simulink model "csec_keyconfig_s32k14x"  (Simulink 9.0)
settings: Solver=FixedStepDiscrete  StartTime=0.0  StopTime=10.0  FixedStep=0.1  RelTol=1e-3  EnableMultiTasking=on
PreLoadFcn:
  | mbd_s32k_examples_preload_cbk;
InitFcn:
  | mbd_s32k_consistency_checks(bdroot(gcs));
undefined symbols (not defined in the file): LQFP
libraries: mbd_s32k1xx_ec_toolbox x37, simulink x1
Description:
  | This model presents basic usecases for the CSEc driver.
  | 
  | This application demonstrates how to use:
  | - CSEc_Enable block to enable the CSEc module by partitioning the Flash.
  | - CSEc_Compute_M1M2M3 and CSEc_Load_Key block to configure the MASTER_ECU key and the first user key, using the MASTER_ECU key as an authorization.
  | - CSEc_Encrypt and CSEc_Decrypt blocks to encrypt a plain text and decrypt the cipher text using the first user key.
  | - CSEc_Disable block to disable the CSEc module by erasing of all configured keys (including the MASTER_ECU key) using a Challenge-Authentication process.
  |   This will place the part back into factory status (the CSEc module needs to be enabled again).
  | 
  | Output:
  | - RGB LED is green if the encrypted plain text is the same as the one decrypted.
  | - RGB LED is red if the user key 1 couldn't be updated. This can happened if the counter wasn't increased.
  | - RGB LED is yellow if the CSEc module was disabled successfully.
  | 
  | Note:
  | - The first time when running the example on the board, or after a key erase, this example should be ran from RAM. This is needed because the Flash is partitioned to enable the CSEc module.
  | - The user keys are non-volatile. Once the key was loaded using this example, in order to update it, the counter should be increased.
  | - To disable CSEc module (erase all user keys) set disable_csec_flag to 1.
  | 
  | HW prerequisite:
  | - S32K142EVB-Q100 / S32K144EVB-Q100 / S32K146EVB-Q144 / S32K148EVB-Q144
PostSaveFcn:
  | mbd_s32k_examples_postsave_cbk;
settings Model: Creator=NXP MBDT Team  LastModifiedBy=nxf35172
settings DataIOCC: ExternalInput=off  InitialState=off  LimitDataPoints=on  SaveOutput=off  SignalLogging=off  SaveTime=off
settings OptimizationCC: DefaultParameterBehavior=Inlined  LifeSpan=1
settings DebuggingCC: SolverPrmCheckMsg=warning  InheritedTsInSrcMsg=none  SingleTaskRateTransMsg=error  UnconnectedInputMsg=error  UnconnectedOutputMsg=error  UnconnectedLineMsg=error  AllowSymbolicDim=off  UnknownTsInhSupMsg=error  StateNameClashWarn=warning
settings HardwareCC: ProdLargestAtomicInteger=Long  ProdLargestAtomicFloat=Double  ProdEndianess=LittleEndian  ProdHWDeviceType=ARM Compatible->ARM Cortex
settings SFSimCC: MATLABDynamicMemAlloc=off
settings RTWCC: SystemTargetFile=mbd_s32k.tlc  MakeCommand=mbd_s32k_make_rtw COPY_MDLREF_INCLUDES=0  TemplateMakefile=mbd_s32k.tmf  Description=Model Based Design Toolbox S32K14x Code Generation Target
settings CodeAppCC: IgnoreCustomStorageClasses=off
settings STFCustomTargetCC: CombineOutputUpdateFcns=on  ERTCustomFileBanners=on  SupportContinuousTime=off  SupportNonInlinedSFcns=off  RemoveResetFunc=on  MATLABClassNameForMDSCustomization=Simulink.SoftwareTarget.ERTCustomization  GRTInterface=off  SystemTargetFile=mbd_s32k14.tlc
settings ERTTargetCC: MultiwordLength=2048  ParMdlRefBuildCompliant=off  CompOptLevelCompliant=off  ConcurrentExecutionCompliant=off  ModelStepFunctionPrototypeControlCompliant=off  CPPClassGenCompliant=off  UseToolchainInfoCompliant=off  InlinedParameterPlacement=NonHierarchical  ERTCustomFileTemplate=example_file_process.tlc  ConvertIfToSwitch=off  SuppressUnreachableDefaultCases=off

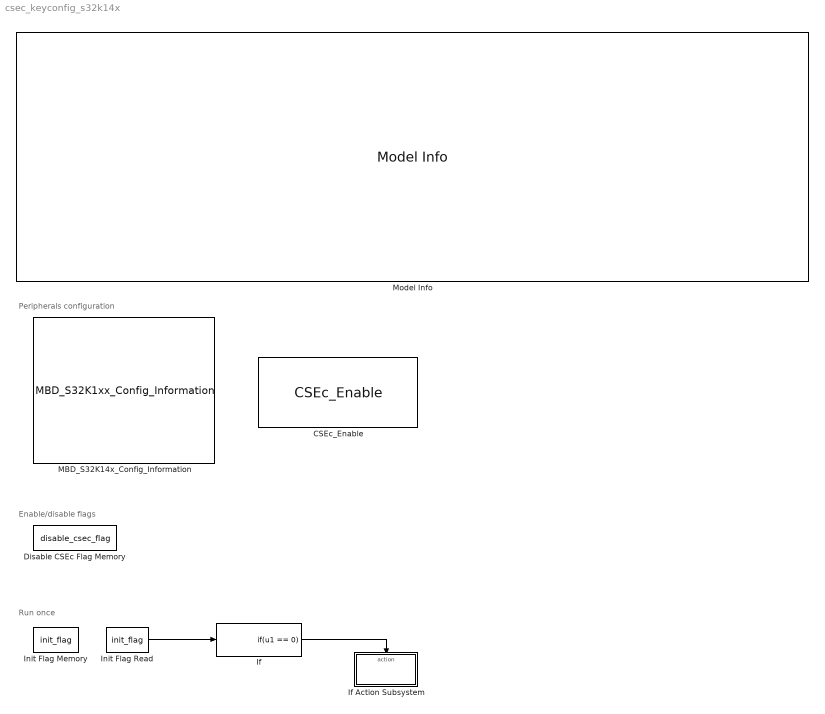
== system csec_keyconfig_s32k14x ==
  note: Enable/disable flags
  note: Peripherals configuration
  note: Run once
  CSEc_Enable : mbd_s32k1xx_ec_toolbox/Core and System Blocks/CSEc Blocks/CSEc_Enable  csec_num_user_keys=20 keys
  Disable CSEc Flag Memory : DataStoreMemory  DataStoreName=disable_csec_flag  ReadBeforeWriteMsg=warning  WriteAfterWriteMsg=warning  WriteAfterReadMsg=warning  InitialValue=1  ShowAdditionalParam=off  OutDataTypeStr=uint32
  If : If  IfExpression=u1 == 0  ShowElse=off
  If Action Subsystem : Subsystem  TreatAsAtomicUnit=on
  Init Flag Memory : DataStoreMemory  DataStoreName=init_flag  ReadBeforeWriteMsg=warning  WriteAfterWriteMsg=warning  WriteAfterReadMsg=warning  ShowAdditionalParam=off  OutDataTypeStr=uint32
  Init Flag Read : DataStoreRead  DataStoreName=init_flag
  MBD_S32K14x_Config_Information : mbd_s32k1xx_ec_toolbox/MBD_S32K1xx_Config_Information  mbdt_ver=0  disp_str=|  config_params=[]  mcu_target_name=S32K144  mcu_target_package=64-LQFP  mcu_target_sram_size=64KB  mcu_system_clock_freq=80  mcu_xtal_freq=External 8  mcu_steptick_timer=LPIT Channel 0  mcu_steptick_prio=15  ds_import_enable=on  target_compiler=GCC  target_memory=SRAM  gcc_target_compile_opts=-mcpu=cortex-m4 -mthumb -mfloat-abi=hard -mfpu=fpv4-sp-d16 -O1 -g -gstrict-dwarf  gcc_target_assemble_opts=-mcpu=cortex-m4 -mthumb -mfloat-abi=hard -mfpu=fpv4-sp-d16 -g  gcc_target_link_opts=-mcpu=cortex-m4 -mthumb -mfloat-abi=hard -mfpu=fpv4-sp-d16  gcc_target_default_lcf=on  gcc_target_user_lcf=S32K144_64_ram.ld  ghs_target_compile_opts=-cpu=cortexm4f -thumb -DARM_MATH_CM4 -fpu=vfpv4_d16 -fsingle -Ogeneral -Wundef -Wimplicit-int -Wshadow -Wtrigraphs --no_commons --gnu_asm -gnu99 -gdwarf-2 -G  ghs_target_assemble_opts=-cpu=cortexm4f -fpu=vfpv4_d16  ghs_target_link_opts=-cpu=cortexm4f -thumb -fpu=vfpv4_d16  ghs_target_default_lcf=off  ghs_target_user_lcf=S32K144_64_ram.ld  iar_target_compile_opts=--cpu=Cortex-M4F --thumb --fpu=VFPv4_sp -Ol -e --debug --dlib_config normal  iar_target_assemble_opts=--cpu Cortex-M4F --thumb --fpu VFPv4_sp  iar_target_link_opts=--no_exceptions --vfe --inline  iar_target_default_lcf=off  iar_target_user_lcf=S32K144_64_ram.icf  pil_download_enable=off  rbl_download_enable=on  rbl_start_delay=5000000  rbl_download_interface=Serial  rbl_restart_request=on  rbl_com_port=Custom  rbl_com_port_custom=COM1  pil_download_rate=57600  pil_opensda_drive=Custom  pil_opensda_drive_custom=D  pil_uart_instance=0  pil_uart_rx=PTA2: [LPUART0_RX | Receive]  pil_uart_tx=PTA3: [LPUART0_TX | Transmit]  FTM_PWM_PcrCheckEnDis=on  FTM_Input_Edge_Inputs_PcrCheckEnDis=on  FTM_Dual_Edge_Inputs_PcrCheckEnDis=on  FTM_Quadrature_Inputs_PcrCheckEnDis=on  FTM_Hall_Sensor_Inputs_PcrCheckEnDis=on  LPTMR_PcrCheckEnDis=on  PIT_PcrCheckEnDis=on  RTC_PcrCheckEnDis=on  FlexCAN_PcrCheckEnDis=on  LIN_PcrCheckEnDis=on  FlexIO_PcrCheckEnDis=on  LPI2C_PcrCheckEnDis=on  LPSPI_PcrCheckEnDis=on  LPUART_PcrCheckEnDis=on  CMP_PcrCheckEnDis=on  GPIO_OutputPcrCheckEnDis=on  GPIO_InputPcrCheckEnDis=on  SBC_PcrCheckEnDis=on  AMMCLIB_PcrCheckEnDis=on  FM_PcrCheckEnDis=on  Profile_PcrCheckEnDis=on  ConfigParams_PcrCheckEnDis=on  ModelRef_PcrCheckEnDis=on  PDB0_PcrCheckEnDis=on  CSEc_PcrCheckEnDis=on  eDMA_PcrCheckEnDis=on  ADC_PcrCheckEnDis=on  WDOG_PcrCheckEnDis=on
      | Target : S32K144-64KB_SRAM
      | Package : 100-pin
      | System clock : 80 MHz
      | XTAL clock : External 8 MHz
      | Compiler : GCC
      | Target Type : SRAM
      | Download Code after build : (COM43, 57600)
      | Step Tick Interrupt Priority : 15
  Model Info : simulink/Model-Wide Utilities/Model Info  Frame=off  DisplayStringWithTags=|  HorizontalTextAlignment=Left  LeftAlignmentValue=0.02
      | Model Name: %<ModelName>
      | 
      | Description: %<Description>
  wires:
  If/1 -> If Action Subsystem/Action
  Init Flag Read/1 -> If/1

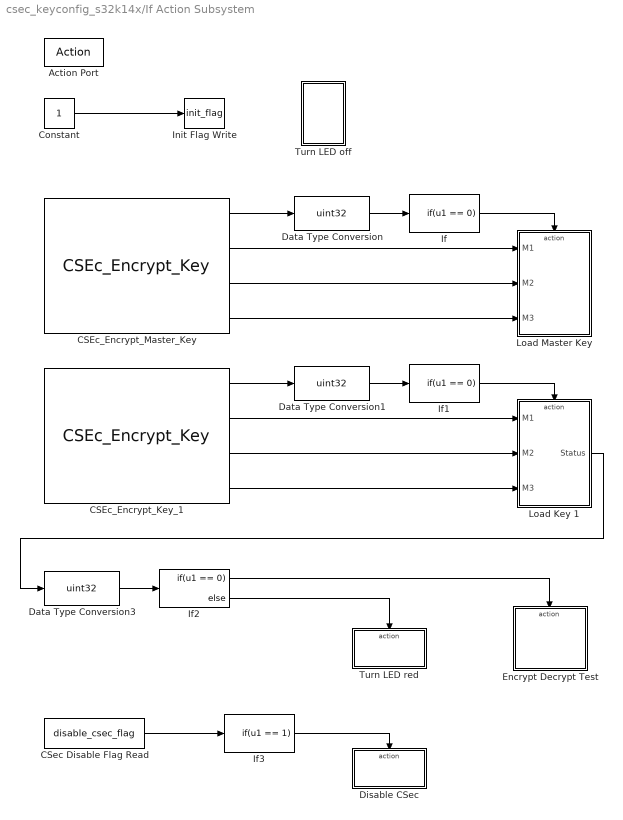
== system csec_keyconfig_s32k14x/If Action Subsystem ==
  Action Port : ActionPort
  CSEc_Encrypt_Key_1 : mbd_s32k1xx_ec_toolbox/Core and System Blocks/CSEc Blocks/CSEc_Encrypt_Key  Priority=3  csec_key_id=KEY_1  csec_key={'0x00', '0x01', '0x02', '0x03', '0x04', '0x05', '0x06', '0x07', '0x08', '0x09', '0x0a', '0x0b', '0x0c', '0x0d', '0x0e', '0x0f'}  csec_auth_key_id=MASTER_ECU  csec_auth_key={'0x00', '0x01', '0x02', '0x03', '0x04', '0x05', '0x06', '0x07', '0x08', '0x09', '0x0a', '0x0b', '0x0c', '0x0d', '0x0e', '0x0f'}  csec_counter=1
  CSEc_Encrypt_Master_Key : mbd_s32k1xx_ec_toolbox/Core and System Blocks/CSEc Blocks/CSEc_Encrypt_Key  Priority=2  csec_key_id=MASTER_ECU  csec_key={'0x00', '0x01', '0x02', '0x03', '0x04', '0x05', '0x06', '0x07', '0x08', '0x09', '0x0a', '0x0b', '0x0c', '0x0d', '0x0e', '0x0f'}  csec_auth_key_id=MASTER_ECU  csec_auth_key={'0xff', '0xff', '0xff', '0xff', '0xff', '0xff', '0xff', '0xff', '0xff', '0xff', '0xff', '0xff', '0xff', '0xff', '0xff', '0xff'}  csec_counter=1
  CSec Disable Flag Read : DataStoreRead  DataStoreName=disable_csec_flag
  Constant : Constant  OutDataTypeStr=uint32
  Data Type Conversion : DataTypeConversion  OutDataTypeStr=uint32
  Data Type Conversion1 : DataTypeConversion  OutDataTypeStr=uint32
  Data Type Conversion3 : DataTypeConversion  OutDataTypeStr=uint32
  Disable CSec : Subsystem  Priority=5  TreatAsAtomicUnit=on
  Encrypt Decrypt Test : Subsystem
  If : If  IfExpression=u1 == 0  ShowElse=off
  If1 : If  IfExpression=u1 == 0  ShowElse=off
  If2 : If  IfExpression=u1 == 0
  If3 : If  IfExpression=u1 == 1  ShowElse=off
  Init Flag Write : DataStoreWrite  DataStoreName=init_flag
  Load Key 1 : Subsystem  Priority=3
  Load Master Key : Subsystem  Priority=2
  Turn LED off : Subsystem  Priority=1
  Turn LED red : Subsystem  Priority=4  TreatAsAtomicUnit=on
  wires:
  Constant/1 -> Init Flag Write/1
  If3/1 -> Disable CSec/Action
  CSec Disable Flag Read/1 -> If3/1
  CSEc_Encrypt_Master_Key/2 -> Load Master Key/1(M1)
  CSEc_Encrypt_Master_Key/3 -> Load Master Key/2(M2)
  CSEc_Encrypt_Master_Key/4 -> Load Master Key/3(M3)
  CSEc_Encrypt_Key_1/2 -> Load Key 1/1(M1)
  CSEc_Encrypt_Key_1/3 -> Load Key 1/2(M2)
  CSEc_Encrypt_Key_1/4 -> Load Key 1/3(M3)
  If1/1 -> Load Key 1/Action
  If/1 -> Load Master Key/Action
  CSEc_Encrypt_Master_Key/1 -> Data Type Conversion/1
  Data Type Conversion/1 -> If/1
  Data Type Conversion1/1 -> If1/1
  CSEc_Encrypt_Key_1/1 -> Data Type Conversion1/1
  If2/1 -> Encrypt Decrypt Test/Action
  Data Type Conversion3/1 -> If2/1
  Load Key 1/1(Status) -> Data Type Conversion3/1
  If2/2 -> Turn LED red/Action

== system csec_keyconfig_s32k14x/If Action Subsystem/Disable CSec ==
  Action Port : ActionPort
  CSEc_Disable : mbd_s32k1xx_ec_toolbox/Core and System Blocks/CSEc Blocks/CSEc_Disable  csec_master_key={'0x00', '0x01', '0x02', '0x03', '0x04', '0x05', '0x06', '0x07', '0x08', '0x09', '0x0a', '0x0b', '0x0c', '0x0d', '0x0e', '0x0f'}
  If3 : If  IfExpression=u1 == 1  ShowElse=off
  Turn LED yellow : Subsystem  Priority=4  TreatAsAtomicUnit=on
  wires:
  If3/1 -> Turn LED yellow/Action
  CSEc_Disable/1 -> If3/1

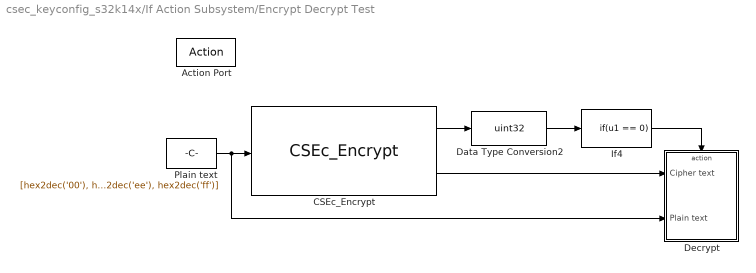
== system csec_keyconfig_s32k14x/If Action Subsystem/Encrypt Decrypt Test ==
  Action Port : ActionPort
  CSEc_Encrypt : mbd_s32k1xx_ec_toolbox/Core and System Blocks/CSEc Blocks/CSEc_Encrypt  Priority=4  csec_mode=Electronic Codebook (ECB)  csec_key_id=KEY_1  csec_timeout=0
  Data Type Conversion2 : DataTypeConversion  OutDataTypeStr=uint32
  Decrypt : Subsystem  Priority=4
  If4 : If  IfExpression=u1 == 0  ShowElse=off
  Plain text : Constant  Value=[hex2dec('00'), hex2dec('11'), hex2dec('22'), hex2dec('33'), hex2dec('44'), hex2dec('55'), hex2dec('66'), hex2dec('77'), hex2dec('88'), hex2dec('99'), hex2dec('aa'), hex2dec('bb'), hex2dec('cc'), hex2dec('dd'), hex2dec('ee'), hex2dec('ff')]  OutDataTypeStr=uint8
  wires:
  CSEc_Encrypt/2 -> Decrypt/1(Cipher text)
  If4/1 -> Decrypt/Action
  CSEc_Encrypt/1 -> Data Type Conversion2/1
  Data Type Conversion2/1 -> If4/1
  Plain text/1 -> CSEc_Encrypt/1, Decrypt/2(Plain text)

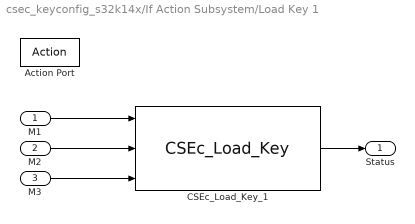
== system csec_keyconfig_s32k14x/If Action Subsystem/Load Key 1 ==
  M1 : Inport
  M2 : Inport  Port=2
  M3 : Inport  Port=3
  Action Port : ActionPort
  CSEc_Load_Key_1 : mbd_s32k1xx_ec_toolbox/Core and System Blocks/CSEc Blocks/CSEc_Load_Key  csec_key_id=KEY_1  csec_load_plain_key=off
  Status : Outport
  wires:
  M1/1 -> CSEc_Load_Key_1/1
  M2/1 -> CSEc_Load_Key_1/2
  M3/1 -> CSEc_Load_Key_1/3
  CSEc_Load_Key_1/1 -> Status/1

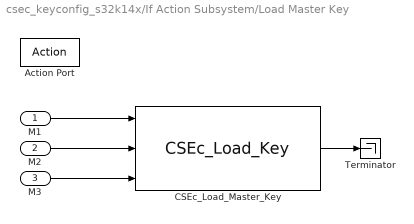
== system csec_keyconfig_s32k14x/If Action Subsystem/Load Master Key ==
  M1 : Inport
  M2 : Inport  Port=2
  M3 : Inport  Port=3
  Action Port : ActionPort
  CSEc_Load_Master_Key : mbd_s32k1xx_ec_toolbox/Core and System Blocks/CSEc Blocks/CSEc_Load_Key  csec_key_id=MASTER_ECU  csec_load_plain_key=off
  Terminator : Terminator
  wires:
  M1/1 -> CSEc_Load_Master_Key/1
  M2/1 -> CSEc_Load_Master_Key/2
  M3/1 -> CSEc_Load_Master_Key/3
  CSEc_Load_Master_Key/1 -> Terminator/1

== system csec_keyconfig_s32k14x/If Action Subsystem/Turn LED off ==
  Blue LED off : Subsystem
      mask Display: disp('Blue LED off');
  Green LED off : Subsystem
      mask Display: disp('Green LED off');
  Red LED off : Subsystem
      mask Display: disp('Red LED off');

== system csec_keyconfig_s32k14x/If Action Subsystem/Turn LED red ==
  Action Port : ActionPort
  Red LED on : Subsystem
      mask Display: disp('Red LED on');

== system csec_keyconfig_s32k14x/If Action Subsystem/Disable CSec/Turn LED yellow ==
  Action Port : ActionPort
  Green LED on : Subsystem
      mask Display: disp('Green LED on');
  Red LED on : Subsystem
      mask Display: disp('Red LED on');

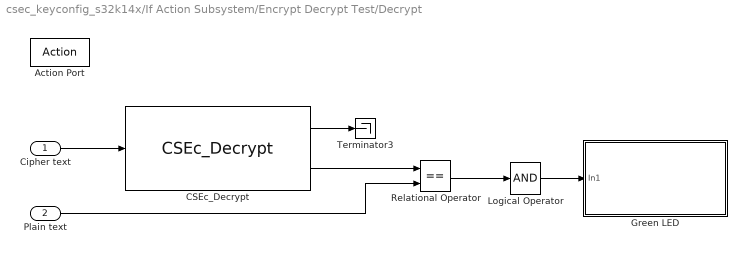
== system csec_keyconfig_s32k14x/If Action Subsystem/Encrypt Decrypt Test/Decrypt ==
  Cipher text : Inport
  Plain text : Inport  Port=2
  Action Port : ActionPort
  CSEc_Decrypt : mbd_s32k1xx_ec_toolbox/Core and System Blocks/CSEc Blocks/CSEc_Decrypt  Priority=3  csec_mode=Electronic Codebook (ECB)  csec_key_id=KEY_1  csec_timeout=1
  Green LED : Subsystem  Variant=on
      mask Display:
      | disp('Green LED');
      | port_label('input',1,'out')
  Logical Operator : Logic  Inputs=1  AllPortsSameDT=off  OutDataTypeStr=boolean
  Relational Operator : RelationalOperator  Operator===  OutDataTypeStr=boolean  RndMeth=Nearest
  Terminator3 : Terminator
  wires:
  Cipher text/1 -> CSEc_Decrypt/1
  CSEc_Decrypt/1 -> Terminator3/1
  CSEc_Decrypt/2 -> Relational Operator/1
  Logical Operator/1 -> Green LED/1(In1)
  Relational Operator/1 -> Logical Operator/1
  Plain text/1 -> Relational Operator/2

== system csec_keyconfig_s32k14x/If Action Subsystem/Turn LED off/Blue LED off ==
  Blue LED : Subsystem  Variant=on
      mask Display:
      | disp('Blue LED');
      | port_label('input',1,'out')
  Constant : Constant  Value=0  OutDataTypeStr=boolean
  wires:
  Constant/1 -> Blue LED/1(In1)

== system csec_keyconfig_s32k14x/If Action Subsystem/Turn LED off/Green LED off ==
  Constant : Constant  Value=0  OutDataTypeStr=boolean
  Green LED : Subsystem  Variant=on
      mask Display:
      | disp('Green LED');
      | port_label('input',1,'out')
  wires:
  Constant/1 -> Green LED/1(In1)

== system csec_keyconfig_s32k14x/If Action Subsystem/Turn LED off/Red LED off ==
  Constant : Constant  Value=0  OutDataTypeStr=boolean
  Red LED : Subsystem  Variant=on
      mask Display:
      | disp('Red LED');
      | port_label('input',1,'out')
  wires:
  Constant/1 -> Red LED/1(In1)

== system csec_keyconfig_s32k14x/If Action Subsystem/Turn LED red/Red LED on ==
  Constant : Constant  OutDataTypeStr=boolean
  Red LED : Subsystem  Variant=on
      mask Display:
      | disp('Red LED');
      | port_label('input',1,'out')
  wires:
  Constant/1 -> Red LED/1(In1)

== system csec_keyconfig_s32k14x/If Action Subsystem/Disable CSec/Turn LED yellow/Green LED on ==
  Constant : Constant  OutDataTypeStr=boolean
  Green LED : Subsystem  Variant=on
      mask Display:
      | disp('Green LED');
      | port_label('input',1,'out')
  wires:
  Constant/1 -> Green LED/1(In1)

== system csec_keyconfig_s32k14x/If Action Subsystem/Disable CSec/Turn LED yellow/Red LED on ==
  Constant : Constant  OutDataTypeStr=boolean
  Red LED : Subsystem  Variant=on
      mask Display:
      | disp('Red LED');
      | port_label('input',1,'out')
  wires:
  Constant/1 -> Red LED/1(In1)

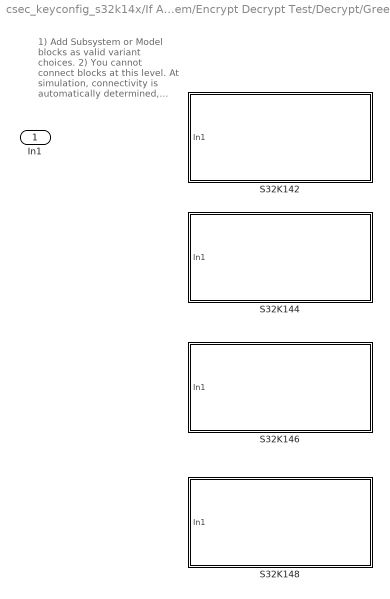
== system csec_keyconfig_s32k14x/If Action Subsystem/Encrypt Decrypt Test/Decrypt/Green LED ==
  note: 1) Add Subsystem or Model blocks as valid variant choices.
      | 2) You cannot connect blocks at this level. At simulation, connectivity is automatically
      | determined, based on the active variant and port name matching.
  In1 : Inport
  S32K142 : Subsystem  VariantControl=VSS_S32k142
  S32K144 : Subsystem  VariantControl=VSS_S32k144
  S32K146 : Subsystem  VariantControl=VSS_S32k146
  S32K148 : Subsystem  VariantControl=VSS_S32k148

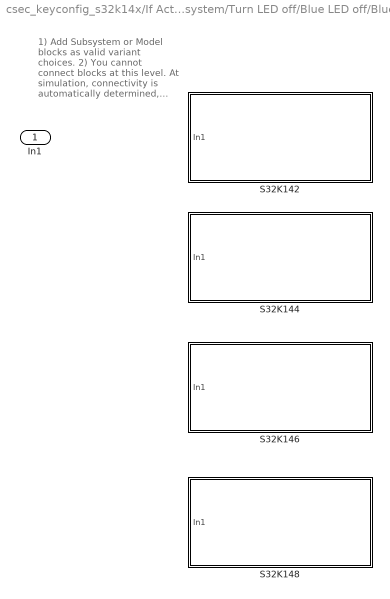
== system csec_keyconfig_s32k14x/If Action Subsystem/Turn LED off/Blue LED off/Blue LED ==
  note: 1) Add Subsystem or Model blocks as valid variant choices.
      | 2) You cannot connect blocks at this level. At simulation, connectivity is automatically
      | determined, based on the active variant and port name matching.
  In1 : Inport
  S32K142 : Subsystem  VariantControl=VSS_S32k142
  S32K144 : Subsystem  VariantControl=VSS_S32k144
  S32K146 : Subsystem  VariantControl=VSS_S32k146
  S32K148 : Subsystem  VariantControl=VSS_S32k148

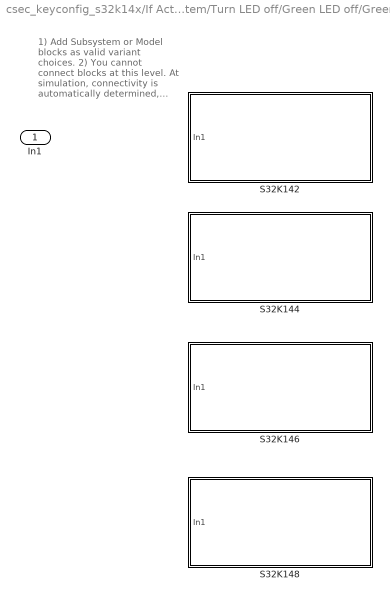
== system csec_keyconfig_s32k14x/If Action Subsystem/Turn LED off/Green LED off/Green LED ==
  note: 1) Add Subsystem or Model blocks as valid variant choices.
      | 2) You cannot connect blocks at this level. At simulation, connectivity is automatically
      | determined, based on the active variant and port name matching.
  In1 : Inport
  S32K142 : Subsystem  VariantControl=VSS_S32k142
  S32K144 : Subsystem  VariantControl=VSS_S32k144
  S32K146 : Subsystem  VariantControl=VSS_S32k146
  S32K148 : Subsystem  VariantControl=VSS_S32k148

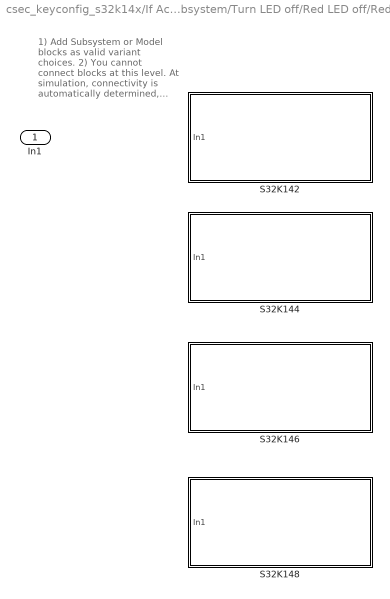
== system csec_keyconfig_s32k14x/If Action Subsystem/Turn LED off/Red LED off/Red LED ==
  note: 1) Add Subsystem or Model blocks as valid variant choices.
      | 2) You cannot connect blocks at this level. At simulation, connectivity is automatically
      | determined, based on the active variant and port name matching.
  In1 : Inport
  S32K142 : Subsystem  VariantControl=VSS_S32k142
  S32K144 : Subsystem  VariantControl=VSS_S32k144
  S32K146 : Subsystem  VariantControl=VSS_S32k146
  S32K148 : Subsystem  VariantControl=VSS_S32k148

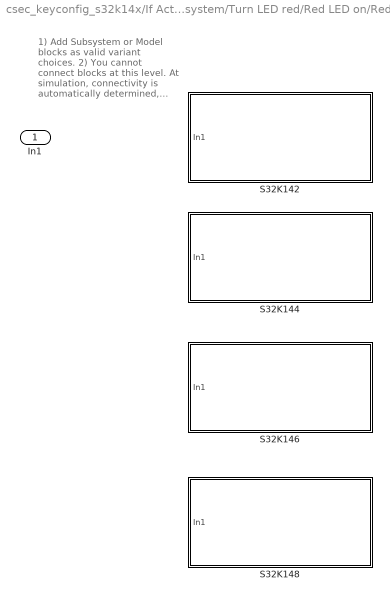
== system csec_keyconfig_s32k14x/If Action Subsystem/Turn LED red/Red LED on/Red LED ==
  note: 1) Add Subsystem or Model blocks as valid variant choices.
      | 2) You cannot connect blocks at this level. At simulation, connectivity is automatically
      | determined, based on the active variant and port name matching.
  In1 : Inport
  S32K142 : Subsystem  VariantControl=VSS_S32k142
  S32K144 : Subsystem  VariantControl=VSS_S32k144
  S32K146 : Subsystem  VariantControl=VSS_S32k146
  S32K148 : Subsystem  VariantControl=VSS_S32k148

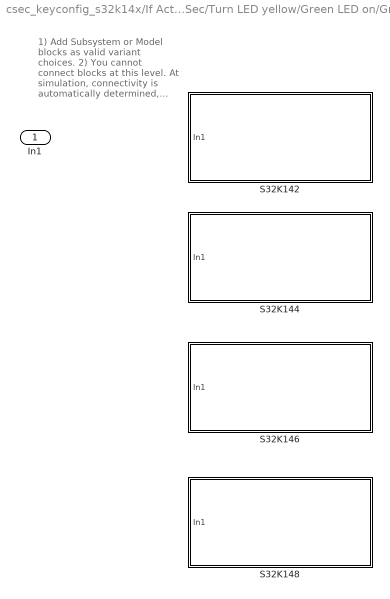
== system csec_keyconfig_s32k14x/If Action Subsystem/Disable CSec/Turn LED yellow/Green LED on/Green LED ==
  note: 1) Add Subsystem or Model blocks as valid variant choices.
      | 2) You cannot connect blocks at this level. At simulation, connectivity is automatically
      | determined, based on the active variant and port name matching.
  In1 : Inport
  S32K142 : Subsystem  VariantControl=VSS_S32k142
  S32K144 : Subsystem  VariantControl=VSS_S32k144
  S32K146 : Subsystem  VariantControl=VSS_S32k146
  S32K148 : Subsystem  VariantControl=VSS_S32k148

== system csec_keyconfig_s32k14x/If Action Subsystem/Disable CSec/Turn LED yellow/Red LED on/Red LED ==
  note: 1) Add Subsystem or Model blocks as valid variant choices.
      | 2) You cannot connect blocks at this level. At simulation, connectivity is automatically
      | determined, based on the active variant and port name matching.
  In1 : Inport
  S32K142 : Subsystem  VariantControl=VSS_S32k142
  S32K144 : Subsystem  VariantControl=VSS_S32k144
  S32K146 : Subsystem  VariantControl=VSS_S32k146
  S32K148 : Subsystem  VariantControl=VSS_S32k148

== system csec_keyconfig_s32k14x/If Action Subsystem/Encrypt Decrypt Test/Decrypt/Green LED/S32K142 ==
  In1 : Inport
  Green_LED : mbd_s32k1xx_ec_toolbox/GPIO Blocks/Digital_Output  gpio_pin=PTD16: [PTD16 | Port D I/O]  init_val=Low  drive_strength=Low
  wires:
  In1/1 -> Green_LED/1

== system csec_keyconfig_s32k14x/If Action Subsystem/Encrypt Decrypt Test/Decrypt/Green LED/S32K144 ==
  In1 : Inport
  Green_LED : mbd_s32k1xx_ec_toolbox/GPIO Blocks/Digital_Output  gpio_pin=PTD16: [PTD16 | Port D I/O]  init_val=Low  drive_strength=Low
  Logical Operator : Logic  Operator=NOT  AllPortsSameDT=off  OutDataTypeStr=boolean
  wires:
  In1/1 -> Logical Operator/1
  Logical Operator/1 -> Green_LED/1

== system csec_keyconfig_s32k14x/If Action Subsystem/Encrypt Decrypt Test/Decrypt/Green LED/S32K146 ==
  In1 : Inport
  Green_LED : mbd_s32k1xx_ec_toolbox/GPIO Blocks/Digital_Output  gpio_pin=PTD16: [PTD16 | Port D I/O]  init_val=Low  drive_strength=Low
  wires:
  In1/1 -> Green_LED/1

== system csec_keyconfig_s32k14x/If Action Subsystem/Encrypt Decrypt Test/Decrypt/Green LED/S32K148 ==
  In1 : Inport
  Green_LED : mbd_s32k1xx_ec_toolbox/GPIO Blocks/Digital_Output  gpio_pin=PTE22: [PTE22 | Port E I/O]  init_val=Low  drive_strength=Low
  wires:
  In1/1 -> Green_LED/1

== system csec_keyconfig_s32k14x/If Action Subsystem/Turn LED off/Blue LED off/Blue LED/S32K142 ==
  In1 : Inport
  Blue_LED : mbd_s32k1xx_ec_toolbox/GPIO Blocks/Digital_Output  gpio_pin=PTD0: [PTD0 | Port D I/O]  init_val=Low  drive_strength=Low
  wires:
  In1/1 -> Blue_LED/1

== system csec_keyconfig_s32k14x/If Action Subsystem/Turn LED off/Blue LED off/Blue LED/S32K144 ==
  In1 : Inport
  Blue_LED : mbd_s32k1xx_ec_toolbox/GPIO Blocks/Digital_Output  gpio_pin=PTD0: [PTD0 | Port D I/O]  init_val=Low  drive_strength=Low
  Logical Operator : Logic  Operator=NOT  AllPortsSameDT=off  OutDataTypeStr=boolean
  wires:
  In1/1 -> Logical Operator/1
  Logical Operator/1 -> Blue_LED/1

== system csec_keyconfig_s32k14x/If Action Subsystem/Turn LED off/Blue LED off/Blue LED/S32K146 ==
  In1 : Inport
  Blue_LED : mbd_s32k1xx_ec_toolbox/GPIO Blocks/Digital_Output  gpio_pin=PTD0: [PTD0 | Port D I/O]  init_val=Low  drive_strength=Low
  wires:
  In1/1 -> Blue_LED/1

== system csec_keyconfig_s32k14x/If Action Subsystem/Turn LED off/Blue LED off/Blue LED/S32K148 ==
  In1 : Inport
  Blue_LED : mbd_s32k1xx_ec_toolbox/GPIO Blocks/Digital_Output  gpio_pin=PTE23: [PTE23 | Port E I/O]  init_val=Low  drive_strength=Low
  wires:
  In1/1 -> Blue_LED/1

== system csec_keyconfig_s32k14x/If Action Subsystem/Turn LED off/Green LED off/Green LED/S32K142 ==
  In1 : Inport
  Green_LED : mbd_s32k1xx_ec_toolbox/GPIO Blocks/Digital_Output  gpio_pin=PTD16: [PTD16 | Port D I/O]  init_val=Low  drive_strength=Low
  wires:
  In1/1 -> Green_LED/1

== system csec_keyconfig_s32k14x/If Action Subsystem/Turn LED off/Green LED off/Green LED/S32K144 ==
  In1 : Inport
  Green_LED : mbd_s32k1xx_ec_toolbox/GPIO Blocks/Digital_Output  gpio_pin=PTD16: [PTD16 | Port D I/O]  init_val=Low  drive_strength=Low
  Logical Operator : Logic  Operator=NOT  AllPortsSameDT=off  OutDataTypeStr=boolean
  wires:
  In1/1 -> Logical Operator/1
  Logical Operator/1 -> Green_LED/1

== system csec_keyconfig_s32k14x/If Action Subsystem/Turn LED off/Green LED off/Green LED/S32K146 ==
  In1 : Inport
  Green_LED : mbd_s32k1xx_ec_toolbox/GPIO Blocks/Digital_Output  gpio_pin=PTD16: [PTD16 | Port D I/O]  init_val=Low  drive_strength=Low
  wires:
  In1/1 -> Green_LED/1

== system csec_keyconfig_s32k14x/If Action Subsystem/Turn LED off/Green LED off/Green LED/S32K148 ==
  In1 : Inport
  Green_LED : mbd_s32k1xx_ec_toolbox/GPIO Blocks/Digital_Output  gpio_pin=PTE22: [PTE22 | Port E I/O]  init_val=Low  drive_strength=Low
  wires:
  In1/1 -> Green_LED/1

== system csec_keyconfig_s32k14x/If Action Subsystem/Turn LED off/Red LED off/Red LED/S32K142 ==
  In1 : Inport
  Red_LED : mbd_s32k1xx_ec_toolbox/GPIO Blocks/Digital_Output  gpio_pin=PTD15: [PTD15 | Port D I/O]  init_val=Low  drive_strength=Low
  wires:
  In1/1 -> Red_LED/1

== system csec_keyconfig_s32k14x/If Action Subsystem/Turn LED off/Red LED off/Red LED/S32K144 ==
  In1 : Inport
  Logical Operator : Logic  Operator=NOT  AllPortsSameDT=off  OutDataTypeStr=boolean
  Red_LED : mbd_s32k1xx_ec_toolbox/GPIO Blocks/Digital_Output  gpio_pin=PTD15: [PTD15 | Port D I/O]  init_val=Low  drive_strength=Low
  wires:
  In1/1 -> Logical Operator/1
  Logical Operator/1 -> Red_LED/1

== system csec_keyconfig_s32k14x/If Action Subsystem/Turn LED off/Red LED off/Red LED/S32K146 ==
  In1 : Inport
  Red_LED : mbd_s32k1xx_ec_toolbox/GPIO Blocks/Digital_Output  gpio_pin=PTD15: [PTD15 | Port D I/O]  init_val=Low  drive_strength=Low
  wires:
  In1/1 -> Red_LED/1

== system csec_keyconfig_s32k14x/If Action Subsystem/Turn LED off/Red LED off/Red LED/S32K148 ==
  In1 : Inport
  Red_LED : mbd_s32k1xx_ec_toolbox/GPIO Blocks/Digital_Output  gpio_pin=PTE21: [PTE21 | Port E I/O]  init_val=Low  drive_strength=Low
  wires:
  In1/1 -> Red_LED/1

== system csec_keyconfig_s32k14x/If Action Subsystem/Turn LED red/Red LED on/Red LED/S32K142 ==
  In1 : Inport
  Red_LED : mbd_s32k1xx_ec_toolbox/GPIO Blocks/Digital_Output  gpio_pin=PTD15: [PTD15 | Port D I/O]  init_val=Low  drive_strength=Low
  wires:
  In1/1 -> Red_LED/1

== system csec_keyconfig_s32k14x/If Action Subsystem/Turn LED red/Red LED on/Red LED/S32K144 ==
  In1 : Inport
  Logical Operator : Logic  Operator=NOT  AllPortsSameDT=off  OutDataTypeStr=boolean
  Red_LED : mbd_s32k1xx_ec_toolbox/GPIO Blocks/Digital_Output  gpio_pin=PTD15: [PTD15 | Port D I/O]  init_val=Low  drive_strength=Low
  wires:
  In1/1 -> Logical Operator/1
  Logical Operator/1 -> Red_LED/1

== system csec_keyconfig_s32k14x/If Action Subsystem/Turn LED red/Red LED on/Red LED/S32K146 ==
  In1 : Inport
  Red_LED : mbd_s32k1xx_ec_toolbox/GPIO Blocks/Digital_Output  gpio_pin=PTD15: [PTD15 | Port D I/O]  init_val=Low  drive_strength=Low
  wires:
  In1/1 -> Red_LED/1

== system csec_keyconfig_s32k14x/If Action Subsystem/Turn LED red/Red LED on/Red LED/S32K148 ==
  In1 : Inport
  Red_LED : mbd_s32k1xx_ec_toolbox/GPIO Blocks/Digital_Output  gpio_pin=PTE21: [PTE21 | Port E I/O]  init_val=Low  drive_strength=Low
  wires:
  In1/1 -> Red_LED/1

== system csec_keyconfig_s32k14x/If Action Subsystem/Disable CSec/Turn LED yellow/Green LED on/Green LED/S32K142 ==
  In1 : Inport
  Green_LED : mbd_s32k1xx_ec_toolbox/GPIO Blocks/Digital_Output  gpio_pin=PTD16: [PTD16 | Port D I/O]  init_val=Low  drive_strength=Low
  wires:
  In1/1 -> Green_LED/1

== system csec_keyconfig_s32k14x/If Action Subsystem/Disable CSec/Turn LED yellow/Green LED on/Green LED/S32K144 ==
  In1 : Inport
  Green_LED : mbd_s32k1xx_ec_toolbox/GPIO Blocks/Digital_Output  gpio_pin=PTD16: [PTD16 | Port D I/O]  init_val=Low  drive_strength=Low
  Logical Operator : Logic  Operator=NOT  AllPortsSameDT=off  OutDataTypeStr=boolean
  wires:
  In1/1 -> Logical Operator/1
  Logical Operator/1 -> Green_LED/1

== system csec_keyconfig_s32k14x/If Action Subsystem/Disable CSec/Turn LED yellow/Green LED on/Green LED/S32K146 ==
  In1 : Inport
  Green_LED : mbd_s32k1xx_ec_toolbox/GPIO Blocks/Digital_Output  gpio_pin=PTD16: [PTD16 | Port D I/O]  init_val=Low  drive_strength=Low
  wires:
  In1/1 -> Green_LED/1

== system csec_keyconfig_s32k14x/If Action Subsystem/Disable CSec/Turn LED yellow/Green LED on/Green LED/S32K148 ==
  In1 : Inport
  Green_LED : mbd_s32k1xx_ec_toolbox/GPIO Blocks/Digital_Output  gpio_pin=PTE22: [PTE22 | Port E I/O]  init_val=Low  drive_strength=Low
  wires:
  In1/1 -> Green_LED/1

== system csec_keyconfig_s32k14x/If Action Subsystem/Disable CSec/Turn LED yellow/Red LED on/Red LED/S32K142 ==
  In1 : Inport
  Red_LED : mbd_s32k1xx_ec_toolbox/GPIO Blocks/Digital_Output  gpio_pin=PTD15: [PTD15 | Port D I/O]  init_val=Low  drive_strength=Low
  wires:
  In1/1 -> Red_LED/1

== system csec_keyconfig_s32k14x/If Action Subsystem/Disable CSec/Turn LED yellow/Red LED on/Red LED/S32K144 ==
  In1 : Inport
  Logical Operator : Logic  Operator=NOT  AllPortsSameDT=off  OutDataTypeStr=boolean
  Red_LED : mbd_s32k1xx_ec_toolbox/GPIO Blocks/Digital_Output  gpio_pin=PTD15: [PTD15 | Port D I/O]  init_val=Low  drive_strength=Low
  wires:
  In1/1 -> Logical Operator/1
  Logical Operator/1 -> Red_LED/1

== system csec_keyconfig_s32k14x/If Action Subsystem/Disable CSec/Turn LED yellow/Red LED on/Red LED/S32K146 ==
  In1 : Inport
  Red_LED : mbd_s32k1xx_ec_toolbox/GPIO Blocks/Digital_Output  gpio_pin=PTD15: [PTD15 | Port D I/O]  init_val=Low  drive_strength=Low
  wires:
  In1/1 -> Red_LED/1

== system csec_keyconfig_s32k14x/If Action Subsystem/Disable CSec/Turn LED yellow/Red LED on/Red LED/S32K148 ==
  In1 : Inport
  Red_LED : mbd_s32k1xx_ec_toolbox/GPIO Blocks/Digital_Output  gpio_pin=PTE21: [PTE21 | Port E I/O]  init_val=Low  drive_strength=Low
  wires:
  In1/1 -> Red_LED/1
